simulink model "auto_pilot_udp"  (R2022b)
settings: Solver=FixedStepAuto  StartTime=0.0  StopTime=Inf  FixedStep=0.001  RelTol=1e-3  EnableMultiTasking=on
InitFcn:
  | clear mex
model workspace (MAT data in the model file):
  worldsim_instance : object (value not decoded)
values from neighbouring files (symbols this model uses):
  ACC_Adaptive_D = 0    [AutoPilot_parameters.m]    (also in ap_ini_param.mat; ap_initialModel.sldd = 0.0)
  ACC_Adaptive_I = 0    [AutoPilot_parameters.m]    (also in ap_ini_param.mat; ap_initialModel.sldd = 0.0)
  ACC_Adaptive_P = [5 7.5]    [AutoPilot_parameters.m]    (also in ap_ini_param.mat; ap_initialModel.sldd = 5.0 7.5)
  ACC_Classic_I = 5    [AutoPilot_parameters.m]    (also in ap_ini_param.mat; ap_initialModel.sldd = 5.0)
  ACC_Classic_P = 15    [AutoPilot_parameters.m]    (also in ap_ini_param.mat; ap_initialModel.sldd = 15.0)
  ACC_MaxBrake = 50    [AutoPilot_parameters.m]    (also in ap_ini_param.mat; ap_initialModel.sldd = 50.0)
  ACC_MaxThrottle = 130    [AutoPilot_parameters.m]    (also in ap_ini_param.mat = 80; ap_initialModel.sldd = 130.0)
  ACC_Module_Activity_Flag = 1    [AutoPilot_parameters.m]    (also in ap_ini_param.mat; ap_initialModel.sldd = 1.0)
  ACC_Ready_Speed = 30    [AutoPilot_parameters.m]    (also in ap_ini_param.mat; ap_initialModel.sldd = 30.0)
  ACC_SensorMaxDistance = 250    [AutoPilot_parameters.m]    (also in ap_ini_param.mat = 120; ap_initialModel.sldd = 250.0)
  ACC_Speed_Distance_control = 3    [AutoPilot_parameters.m]    (also in ap_ini_param.mat; ap_initialModel.sldd = 3.0)
  ACC_Speed_Distance_Gain = [0.1 0.15 0.2 0.25]    [AutoPilot_parameters.m]    (also in ap_ini_param.mat; ap_initialModel.sldd = 0.1 0.15 0.2 0.25)
  ADAS_Control_Mode = 1    [AutoPilot_parameters.m]    (also in ap_ini_param.mat; ap_initialModel.sldd = 1.0)
  AEB_Alarm_Freq = 5    [AutoPilot_parameters.m]    (also in ap_ini_param.mat; ap_initialModel.sldd = 5.0)
  AEB_Distance_To_Collision_Brake = 5    [AutoPilot_parameters.m]    (also in ap_ini_param.mat; ap_initialModel.sldd = 5.0)
  AEB_Freq_Hz = Sensor_Freq_worldsim/2    (= 25)    [AutoPilot_parameters.m]    (also in ap_ini_param.mat; ap_initialModel.sldd = 25.0)
  AEB_Gain = [1 1]    [AutoPilot_parameters.m]    (also in ap_ini_param.mat; ap_initialModel.sldd = 1.0 1.0)
  AEB_Gain_set = 60    [AutoPilot_parameters.m]    (also in ap_ini_param.mat; ap_initialModel.sldd = 60.0)
  AEB_Gain_set_mult = 0.03    [AutoPilot_parameters.m]    (also in ap_ini_param.mat; ap_initialModel.sldd)
  AEB_Max_Decel = [8 15]    [AutoPilot_parameters.m]    (also in ap_ini_param.mat; ap_initialModel.sldd = 8.0 15.0)
  AEB_Max_Speed = 150    [AutoPilot_parameters.m]    (also in ap_ini_param.mat = 100; ap_initialModel.sldd = 150.0)
  AEB_Min_Distance_at_Stop = 1    [AutoPilot_parameters.m]    (also in ap_ini_param.mat; ap_initialModel.sldd = 1.0)
  AEB_Module_Activity_Flag = 1    [AutoPilot_parameters.m]    (also in ap_ini_param.mat; ap_initialModel.sldd = 1.0)
  AEB_Pedestrian_type = 68    [AutoPilot_parameters.m]    (also in ap_ini_param.mat; ap_initialModel.sldd = 68.0)
  AEB_Steer_Max = 180    [AutoPilot_parameters.m]    (also in ap_ini_param.mat; ap_initialModel.sldd = 180.0)
  AP_Activity_Flag = 1    [AutoPilot_parameters.m]    (also in ap_ini_param.mat; ap_initialModel.sldd = 1.0)
  AP_D = [0.3 0.3]    [AutoPilot_parameters.m]    (also in ap_ini_param.mat; ap_initialModel.sldd = 0.3 0.3)
  AP_Dyn_Rate_Limiter_Gain = 0.1    [AutoPilot_parameters.m]    (also in ap_ini_param.mat; ap_initialModel.sldd)
  AP_Dyn_Rate_Limiter_Power = 10    [AutoPilot_parameters.m]    (also in ap_ini_param.mat; ap_initialModel.sldd = 10.0)
  AP_Error_Max = 3    [AutoPilot_parameters.m]    (also in ap_ini_param.mat; ap_initialModel.sldd = 3.0)
  AP_Freq_Hz = Sensor_Freq_worldsim    (= 50)    [AutoPilot_parameters.m]    (also in ap_ini_param.mat; ap_initialModel.sldd = 50.0)
  AP_I = [0.05 0.05]    [AutoPilot_parameters.m]    (also in ap_ini_param.mat; ap_initialModel.sldd = 0.05 0.05)
  AP_Max_Error_dydt_Disable = 0.5    [AutoPilot_parameters.m]    (also in ap_ini_param.mat; ap_initialModel.sldd)
  AP_On_Request_Time = 0.01    [AutoPilot_parameters.m]    (also in ap_ini_param.mat; ap_initialModel.sldd)
  AP_P = [0.2 0.2]    [AutoPilot_parameters.m]    (also in ap_ini_param.mat; ap_initialModel.sldd = 0.2 0.2)
  AP_Steer_Error_Max = 0.7    [AutoPilot_parameters.m]    (also in ap_ini_param.mat; ap_initialModel.sldd)
  AP_Steer_Rate_Max_radps = 1    [AutoPilot_parameters.m]    (also in ap_ini_param.mat; ap_initialModel.sldd = 1.0)
  AP_Transition_Rate = 0.5    [AutoPilot_parameters.m]    (also in ap_ini_param.mat; ap_initialModel.sldd)
  butter_a = [1 -1.9911142922 0.991153595869]    [ap_ini_param.mat]    (also in ap_initialModel.sldd = 1.0 -1.9911142922016536 0.99115359586893548)
  butter_a_lka_out = 1.0 -1.5610180758007179 0.641351538057563    [ap_initialModel.sldd]
  butter_b = [9.82591682048e-06 1.9651833641e-05 9.82591682048e-06]    [ap_ini_param.mat]    (also in ap_initialModel.sldd = 9.825916820482009E-6 1.9651833640964018E-5 9.825916820482009)
  butter_b_lka_out = 0.020083365564211246 0.040166731128422492 0.020083365564211246    [ap_initialModel.sldd]
  Lane_Width = 3.7    [AutoPilot_parameters.m]    (also in ap_ini_param.mat; ap_initialModel.sldd)
  LDW_Activity_Flag = 1    [ap_ini_param.mat]    (also in ap_initialModel.sldd = 1.0)
  LDW_Freq_Hz = 50    [ap_ini_param.mat]    (also in ap_initialModel.sldd = 50.0)
  LDW_LaneGap_dydt_Warning = 50    [ap_ini_param.mat]    (also in ap_initialModel.sldd = 50.0)
  LDW_LaneGap_Warning = [0.5 0.25]    [ap_ini_param.mat]    (also in ap_initialModel.sldd = 0.5 0.25)
  LDW_Min_Speed = 60    [ap_ini_param.mat]    (also in ap_initialModel.sldd = 60.0)
  LDW_Steer_Vibration_Amplitude = 5    [ap_ini_param.mat]    (also in ap_initialModel.sldd = 5.0)
  LDW_Steer_Vibration_Freq = 25    [ap_ini_param.mat]    (also in ap_initialModel.sldd = 25.0)
  LKA_Activity_Flag = 1    [ap_ini_param.mat]    (also in ap_initialModel.sldd = 1.0)
  LKA_D = [0.2 0.3]    [ap_ini_param.mat]    (also in ap_initialModel.sldd = 0.2 0.3)
  LKA_Dyn_Rate_Limiter_Gain = 0.1    [ap_ini_param.mat]    (also in ap_initialModel.sldd)
  LKA_Dyn_Rate_Limiter_Power = 10    [ap_ini_param.mat]    (also in ap_initialModel.sldd = 10.0)
  LKA_Error_dydt_Off = 1    [ap_ini_param.mat]    (also in ap_initialModel.sldd = 1.0)
  LKA_Error_Max = 3    [ap_ini_param.mat]    (also in ap_initialModel.sldd = 3.0)
  LKA_Error_Off = 0.5    [ap_ini_param.mat]    (also in ap_initialModel.sldd)
  LKA_Freq_Hz = 50    [ap_ini_param.mat]    (also in ap_initialModel.sldd = 50.0)
  LKA_I = [0.025 0.05]    [ap_ini_param.mat]    (also in ap_initialModel.sldd = 0.025 0.05)
  LKA_Lane_Gap_Activate = [0.25 0.125]    [ap_ini_param.mat]    (also in ap_initialModel.sldd = 0.25 0.125)
  LKA_Lane_Gap_dydt_Activate = 50    [ap_ini_param.mat]    (also in ap_initialModel.sldd = 50.0)
  LKA_Min_Speed = 60    [ap_ini_param.mat]    (also in ap_initialModel.sldd = 60.0)
  LKA_On_Display_Freq = 5    [ap_ini_param.mat]    (also in ap_initialModel.sldd = 5.0)
  LKA_P = [0.1 0.2]    [ap_ini_param.mat]    (also in ap_initialModel.sldd = 0.1 0.2)
  LKA_Steer_Rate_Max_radps = 1    [ap_ini_param.mat]    (also in ap_initialModel.sldd = 1.0)
  No_Target_Display_Value = 0    [AutoPilot_parameters.m]    (also in ap_ini_param.mat; ap_initialModel.sldd = 0.0)
  radar_source = 2    [AutoPilot_parameters.m]    (also in ap_ini_param.mat; ap_initialModel.sldd = 2.0)
  Sensor_Freq_worldsim = 50    [AutoPilot_parameters.m]    (also in ap_ini_param.mat; ap_initialModel.sldd = 50.0; launcher.m)
  stop_number_collisions = 10.0    [ap_initialModel.sldd]    (also in launcher.m = 10)
  stop_speed = 0.001    [ap_initialModel.sldd]    (also in launcher.m)
  stop_time = 12.0    [ap_initialModel.sldd]    (also in launcher.m = 12)
  vehicle_width = 2.2    [AutoPilot_parameters.m]    (also in ap_ini_param.mat = 1.86; ap_initialModel.sldd)
undefined symbols (not defined in the file or in its folder): blockPlatform, HOST, light_brake_center, light_brake_left, light_brake_right
libraries: simulink x103, simwbSfunlib x35, slpidlib x5, viworldsim_lib x5
(part 3 of 5)

== system auto_pilot_udp/OUTPUT/VI-CarRealTime_Outputs2 ==
  Constant : Constant  Value=0
  Gain : Gain  Gain=1/2
  Log_Bus_Creator : BusCreator  Inputs=9
  Log_bus : BusSelector  OutputSignals=VI_CarRealTime:Outputs:chassis_velocities:longitudinal,VI_CarRealTime:Outputs:driver_demands:steering,VI_CarRealTime:Outputs:Wheel:Spindle_Steer:L1,VI_CarRealTime:Outputs:Wheel:Spindle_Steer:R1,VI_CarRealTime:Outputs:driver_demands:throttle,VI_CarRealTime:Outputs:driver_demands:brake,VI_CarRealTime:Outputs:chassis_accelerations:longitudinal,VI_CarRealTime:Outputs:chassis_accelerations:lateral,VI_CarRealTime:Outputs:Steering_System:DriveSim_Steering_Feedback_Torque  OutputAsBus=on
  Scope : Scope  NumInputPorts=2
  Sum : Sum
  Terminator : Terminator
  Terminator1 : Terminator
  VI_CarRealTime.Outputs.Steering_System.DriveSim_Steering_Feedback_Torque : simwbSfunlib/fromRTDBm  varName=VI_CarRealTime.Outputs.Steering_System.DriveSim_Steering_Feedback_Torque  sigDim=[1 1]  sigType=double  sampleTime=[-1 0]  defaultValue=0  hasMapping=0  ptrName=VI_CarRealTime_Outputs_chassis_accelerations_lateral  enumOrAlias=nothing
      settings: SourceProductName=SimWB MLToolkit
  VI_CarRealTime.Outputs.Wheel.Spindle_Steer.L1 : simwbSfunlib/fromRTDBm  varName=VI_CarRealTime.Outputs.Wheel.Spindle_Steer.L1  sigDim=[1 1]  sigType=double  sampleTime=[-1 0]  defaultValue=0  hasMapping=0  ptrName=VI_CarRealTime_Outputs_Wheel_Spindle_Steer_L1  enumOrAlias=nothing
      settings: SourceProductName=SimWB MLToolkit
  VI_CarRealTime.Outputs.Wheel.Spindle_Steer.R1 : simwbSfunlib/fromRTDBm  varName=VI_CarRealTime.Outputs.Wheel.Spindle_Steer.R1  sigDim=[1 1]  sigType=double  sampleTime=[-1 0]  defaultValue=0  hasMapping=0  ptrName=VI_CarRealTime_Outputs_Wheel_Spindle_Steer_R1  enumOrAlias=nothing
      settings: SourceProductName=SimWB MLToolkit
  VI_CarRealTime.Outputs.chassis_accelerations.lateral : simwbSfunlib/fromRTDBm  varName=VI_CarRealTime.Outputs.chassis_accelerations.lateral  sigDim=[1 1]  sigType=double  sampleTime=[-1 0]  defaultValue=0  hasMapping=0  ptrName=VI_CarRealTime_Outputs_chassis_accelerations_longitudinal  enumOrAlias=nothing
      settings: SourceProductName=SimWB MLToolkit
  VI_CarRealTime.Outputs.chassis_accelerations.longitudinal : simwbSfunlib/fromRTDBm  varName=VI_CarRealTime.Outputs.chassis_accelerations.longitudinal  sigDim=[1 1]  sigType=double  sampleTime=[-1 0]  defaultValue=0  hasMapping=0  ptrName=VI_CarRealTime_Outputs_chassis_velocities_longitudinal  enumOrAlias=nothing
      settings: SourceProductName=SimWB MLToolkit
  VI_CarRealTime.Outputs.chassis_velocities.longitudinal : simwbSfunlib/fromRTDBm  varName=VI_CarRealTime.Outputs.chassis_velocities.longitudinal  sigDim=[1 1]  sigType=double  sampleTime=[-1 0]  defaultValue=0  hasMapping=0  ptrName=VI_CarRealTime_Outputs_chassis_velocities_longitudinal  enumOrAlias=nothing
      settings: SourceProductName=SimWB MLToolkit
  VI_CarRealTime.Outputs.driver_demands.brake : simwbSfunlib/fromRTDBm  varName=VI_CarRealTime.Outputs.driver_demands.brake  sigDim=[1 1]  sigType=double  sampleTime=[-1 0]  defaultValue=0  hasMapping=0  ptrName=VI_CarRealTime_Outputs_driver_demands_throttle  enumOrAlias=nothing
      settings: SourceProductName=SimWB MLToolkit
  VI_CarRealTime.Outputs.driver_demands.steering : simwbSfunlib/fromRTDBm  varName=VI_CarRealTime.Outputs.driver_demands.steering  sigDim=[1 1]  sigType=double  sampleTime=[-1 0]  defaultValue=0  hasMapping=0  ptrName=VI_CarRealTime_Outputs_chassis_velocities_longitudinal  enumOrAlias=nothing
      settings: SourceProductName=SimWB MLToolkit
  VI_CarRealTime.Outputs.driver_demands.throttle : simwbSfunlib/fromRTDBm  varName=VI_CarRealTime.Outputs.driver_demands.throttle  sigDim=[1 1]  sigType=double  sampleTime=[-1 0]  defaultValue=0  hasMapping=0  ptrName=VI_CarRealTime_Outputs_driver_demands_steering  enumOrAlias=nothing
      settings: SourceProductName=SimWB MLToolkit
  tag scope: Driver_Brake=global, Driver_Steering=global, Driver_Throttle=global, Front_Axle_Steer=global, Lateral_Accelerations=global, Longitudinal_Accelerations=global, Steering_feedback_torque=global, Vehicle_Speed=global
  wires:
  ? -> Scope/1, [Vehicle_Speed]
  Log_bus/1 -> Terminator/1  "VI_CarRealTime_selection"
  ? -> Scope/2, [Driver_Steering]
  ? -> Sum/1
  ? -> Sum/2
  Sum/1 -> Gain/1
  Gain/1 -> [Front_Axle_Steer]
  ? -> [Driver_Throttle]
  Constant/1 -> [Driver_Brake]
  ? -> Terminator1/1
  ? -> [Longitudinal_Accelerations]
  ? -> [Lateral_Accelerations]
  ? -> [Steering_feedback_torque]
  VI_CarRealTime.Outputs.driver_demands.brake/1 -> Log_Bus_Creator/6  "VI_CarRealTime.Outputs.driver_demands.brake"
  VI_CarRealTime.Outputs.Wheel.Spindle_Steer.L1/1 -> Log_Bus_Creator/3  "VI_CarRealTime.Outputs.Wheel.Spindle_Steer.L1"
  VI_CarRealTime.Outputs.chassis_accelerations.lateral/1 -> Log_Bus_Creator/8  "VI_CarRealTime.Outputs.chassis_accelerations.lateral"
  VI_CarRealTime.Outputs.Steering_System.DriveSim_Steering_Feedback_Torque/1 -> Log_Bus_Creator/9  "VI_CarRealTime.Outputs.Steering_System.DriveSim_Steering_Feedback_Torque"
  VI_CarRealTime.Outputs.chassis_accelerations.longitudinal/1 -> Log_Bus_Creator/7  "VI_CarRealTime.Outputs.chassis_accelerations.longitudinal"
  VI_CarRealTime.Outputs.driver_demands.steering/1 -> Log_Bus_Creator/2  "VI_CarRealTime.Outputs.driver_demands.steering"
  VI_CarRealTime.Outputs.Wheel.Spindle_Steer.R1/1 -> Log_Bus_Creator/4  "VI_CarRealTime.Outputs.Wheel.Spindle_Steer.R1"
  VI_CarRealTime.Outputs.driver_demands.throttle/1 -> Log_Bus_Creator/5  "VI_CarRealTime.Outputs.driver_demands.throttle"
  VI_CarRealTime.Outputs.chassis_velocities.longitudinal/1 -> Log_Bus_Creator/1  "VI_CarRealTime.Outputs.chassis_velocities.longitudinal"
  Log_Bus_Creator/1 -> Log_bus/1

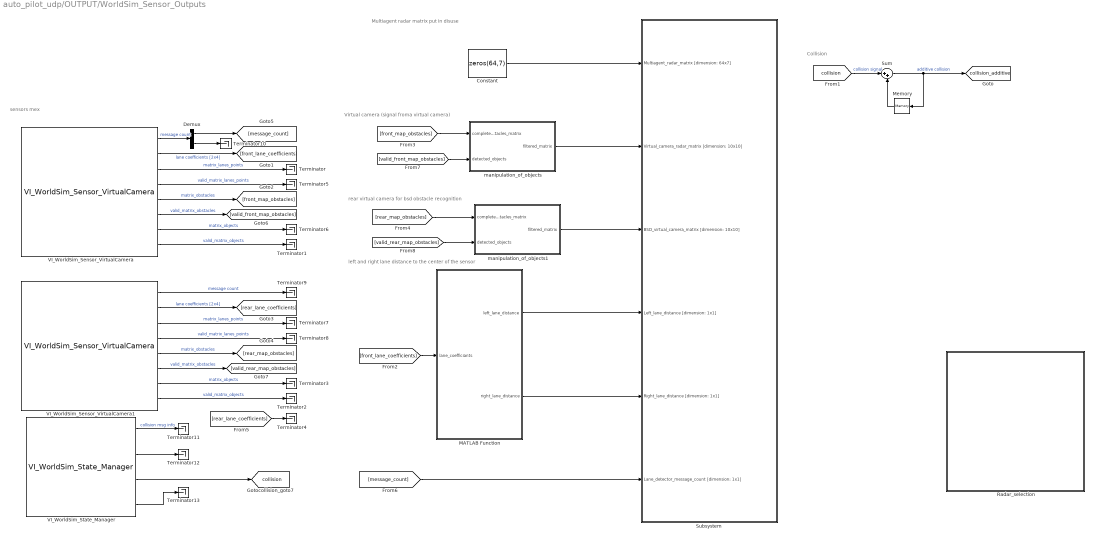
== system auto_pilot_udp/OUTPUT/WorldSim_Sensor_Outputs ==
  note: Collision
  note: left and right lane distance to the center of the sensor
  note: Virtual camera (signal froma virtual camera)
  note: Multiagent radar matrix
      | put in disuse
  note: rear virtual camera for bsd obstacle recognition
  note: sensors mex
  Constant : Constant  Value=zeros(64,7)
  Demux : Demux  Outputs=2
  MATLAB Function : MATLAB Function  TreatAsAtomicUnit=on
  Memory : Memory  InheritSampleTime=on
  Radar_selection : Subsystem
  Subsystem : Subsystem
  Sum : Sum  Inputs=|++
  Terminator{,1..13} (14 alike) : Terminator
  VI_WorldSim_Sensor_VirtualCamera : viworldsim_lib/VI-WorldSim Sensors/VI_WorldSim_Sensor_VirtualCamera  worldsim_endpoint_ip=worldsim_instance.endpoint_ip  worldsim_endpoint_port=worldsim_instance.endpoint_port  worldsim_car_name='ego'  worldsim_sensor_name='Front_VirtualCam'  max_lanes=10  max_obstacles=10  worldsim_verbose=off
  VI_WorldSim_Sensor_VirtualCamera1 : viworldsim_lib/VI-WorldSim Sensors/VI_WorldSim_Sensor_VirtualCamera  worldsim_endpoint_ip=worldsim_instance.endpoint_ip  worldsim_endpoint_port=worldsim_instance.endpoint_port  worldsim_car_name='ego'  worldsim_sensor_name='Rear_VirtualCam'  max_lanes=10  max_obstacles=10  worldsim_verbose=off
  VI_WorldSim_State_Manager : viworldsim_lib/VI-WorldSim Sensors/VI_WorldSim_State_Manager  worldsim_endpoint_ip=worldsim_instance.endpoint_ip  worldsim_endpoint_port=worldsim_instance.endpoint_port  worldsim_car_name='ego'  worldsim_verbose=off
  manipulation_of_objects : MATLAB Function  TreatAsAtomicUnit=on
  manipulation_of_objects1 : MATLAB Function  TreatAsAtomicUnit=on
  tag scope: collision=global, collision_additive=global
  wires:
  Sum/1 -> Memory/1, [collision_additive]  "additive collision"
  [collision] -> Sum/1  "collision signal"
  Memory/1 -> Sum/2
  MATLAB Function/1(left_lane_distance) -> Subsystem/4(Left_lane_distance [dimension: 1x1])
  [message_count] -> Subsystem/6(Lane_detector_message_count [dimension: 1x1])
  manipulation_of_objects1/1(filtered_matrix) -> Subsystem/3(BSD_virtual_camera_matrix [dimension: 10x10])
  manipulation_of_objects/1(filtered_matrix) -> Subsystem/2(Virtual_camera_radar_matrix [dimension: 10x10])
  Constant/1 -> Subsystem/1(Multiagent_radar_matrix [dimension: 64x7])
  [valid_rear_map_obstacles] -> manipulation_of_objects1/2(detected_objects)
  MATLAB Function/2(right_lane_distance) -> Subsystem/5(Right_lane_distance [dimension: 1x1])
  [front_lane_coefficients] -> MATLAB Function/1(lane_coefficiants)
  [rear_map_obstacles] -> manipulation_of_objects1/1(complete_obstacles_matrix)
  [valid_front_map_obstacles] -> manipulation_of_objects/2(detected_objects)
  [front_map_obstacles] -> manipulation_of_objects/1(complete_obstacles_matrix)
  VI_WorldSim_Sensor_VirtualCamera/1 -> Demux/1  "message count"
  VI_WorldSim_State_Manager/1 -> Terminator11/1  "collision msg info"
  VI_WorldSim_Sensor_VirtualCamera/8 -> Terminator1/1  "valid_matrix_objects"
  VI_WorldSim_Sensor_VirtualCamera/5 -> [front_map_obstacles]  "matrix_obstacles"
  VI_WorldSim_Sensor_VirtualCamera/4 -> Terminator5/1  "valid_matrix_lanes_points"
  VI_WorldSim_Sensor_VirtualCamera/6 -> [valid_front_map_obstacles]  "valid_matrix_obstacles"
  VI_WorldSim_Sensor_VirtualCamera1/2 -> [rear_lane_coefficients]  "lane coefficients [2x4]"
  VI_WorldSim_Sensor_VirtualCamera/3 -> Terminator/1  "matrix_lanes_points"
  VI_WorldSim_Sensor_VirtualCamera1/1 -> Terminator9/1  "message count"
  VI_WorldSim_Sensor_VirtualCamera1/7 -> Terminator3/1  "matrix_objects"
  VI_WorldSim_Sensor_VirtualCamera1/8 -> Terminator2/1  "valid_matrix_objects"
  VI_WorldSim_Sensor_VirtualCamera/7 -> Terminator6/1  "matrix_objects"
  VI_WorldSim_Sensor_VirtualCamera/2 -> [front_lane_coefficients]  "lane coefficients [2x4]"
  VI_WorldSim_Sensor_VirtualCamera1/4 -> Terminator8/1  "valid_matrix_lanes_points"
  VI_WorldSim_State_Manager/3 -> [collision]
  VI_WorldSim_Sensor_VirtualCamera1/3 -> Terminator7/1  "matrix_lanes_points"
  [rear_lane_coefficients] -> Terminator4/1
  Demux/2 -> Terminator10/1
  VI_WorldSim_Sensor_VirtualCamera1/5 -> [rear_map_obstacles]  "matrix_obstacles"
  VI_WorldSim_Sensor_VirtualCamera1/6 -> [valid_rear_map_obstacles]  "valid_matrix_obstacles"
  Demux/1 -> [message_count]
  VI_WorldSim_State_Manager/2 -> Terminator12/1
  VI_WorldSim_State_Manager/4 -> Terminator13/1

== system auto_pilot_udp/OUTPUT/rough data reporting ==
  Cast To Double : DataTypeConversion  OutDataTypeStr=double  SaturateOnIntegerOverflow=off  RndMeth=Floor
  Cast To Double1 : DataTypeConversion  OutDataTypeStr=double  SaturateOnIntegerOverflow=off  RndMeth=Floor
  Clock : Clock
  Compare To Constant : simulink/Logic and Bit Operations/Compare To Constant  relop=<=  const=0.0  OutDataTypeStr=boolean
  Compare To Constant1 : simulink/Logic and Bit Operations/Compare To Constant  relop=<=  const=0.0  OutDataTypeStr=boolean
  Compare To Constant2 : simulink/Logic and Bit Operations/Compare To Constant  relop=>  const=0.1  OutDataTypeStr=boolean
  Constant : Constant  Value=0
  Mux : Mux  Inputs=2
  Product : Product
  Scope LDW_Steering_Torque_in_out : Scope
  Sum1 : Sum
  To Workspace : ToWorkspace  VariableName=number_collision  SampleTime=-1
      settings: Save2DSignal=2-D array (concatenate along first dimension)
  To Workspace1 : ToWorkspace  VariableName=longitudinal_accelerations  SampleTime=-1
      settings: Save2DSignal=2-D array (concatenate along first dimension)
  To Workspace2 : ToWorkspace  VariableName=lateral_accelerations  SampleTime=-1
      settings: Save2DSignal=2-D array (concatenate along first dimension)
  To Workspace3 : ToWorkspace  VariableName=crossed_lanes  SampleTime=-1
      settings: Save2DSignal=2-D array (concatenate along first dimension)
  wires:
  Clock/1 -> Compare To Constant2/1
  Compare To Constant1/1 -> Cast To Double1/1
  [Lateral_Accelerations] -> To Workspace2/1
  [LaneGap_right_ws] -> Compare To Constant1/1
  Cast To Double/1 -> Sum1/1
  Compare To Constant2/1 -> Product/2
  [collision_additive] -> To Workspace/1
  Compare To Constant/1 -> Cast To Double/1
  [Longitudinal_Accelerations] -> To Workspace1/1
  [LaneGap_left_ws] -> Compare To Constant/1
  Product/1 -> To Workspace3/1
  Cast To Double1/1 -> Sum1/2
  Sum1/1 -> Product/1
  [Steering_feedback_torque] -> Mux/2
  [LDW_Steering_Torque] -> Mux/1
  Mux/1 -> Scope LDW_Steering_Torque_in_out/1  "LDW_Steering_Torque_in_out"
  Constant/1 -> [LDW_Steering_Torque]

== system auto_pilot_udp/VI-WorldSim Lights Manager/Lights ==
  light_brake_left : Inport
  light_brake_right : Inport  Port=2
  light_brake_center : Inport  Port=3
  Bus Selector : BusSelector  OutputSignals=light_low_beam_left,light_low_beam_right,light_high_beam_left,light_high_beam_right,light_indicator_left,light_indicator_right,light_fog_left,light_fog_right,light_tail_left,light_tail_right,light_brake_left,light_brake_right,light_brake_center,light_reverse,light_daytime
  Default Lights Bus : Subsystem
  LightsBusAssignment : BusAssignment  AssignedSignals=light_brake_left,light_brake_right,light_brake_center
  Mux : Mux  Inputs=15
  Out1 : Outport  VectorParamsAs1DForOutWhenUnconnected=off
  wires:
  LightsBusAssignment/1 -> Bus Selector/1
  Bus Selector/5 -> Mux/5  "<light_indicator_left>"
  Default Lights Bus/1(Out1) -> LightsBusAssignment/1
  Bus Selector/11 -> Mux/11  "<light_brake_left>"
  Bus Selector/10 -> Mux/10  "<light_tail_right>"
  Bus Selector/2 -> Mux/2  "<light_low_beam_right>"
  Bus Selector/9 -> Mux/9  "<light_tail_left>"
  Bus Selector/12 -> Mux/12  "<light_brake_right>"
  Mux/1 -> Out1/1
  Bus Selector/8 -> Mux/8  "<light_fog_right>"
  Bus Selector/14 -> Mux/14  "<light_reverse>"
  Bus Selector/4 -> Mux/4  "<light_high_beam_right>"
  Bus Selector/3 -> Mux/3  "<light_high_beam_left>"
  Bus Selector/15 -> Mux/15  "<light_daytime>"
  Bus Selector/13 -> Mux/13  "<light_brake_center>"
  Bus Selector/6 -> Mux/6  "<light_indicator_right>"
  Bus Selector/1 -> Mux/1  "<light_low_beam_left>"
  Bus Selector/7 -> Mux/7  "<light_fog_left>"
  light_brake_left/1 -> LightsBusAssignment/2
  light_brake_right/1 -> LightsBusAssignment/3
  light_brake_center/1 -> LightsBusAssignment/4

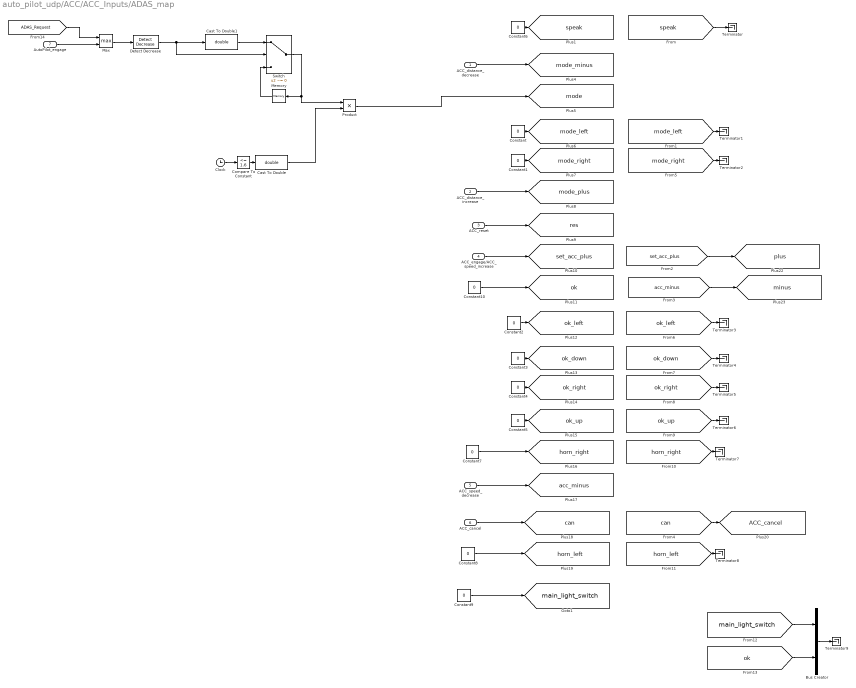
== system auto_pilot_udp/ACC/ACC_Inputs/ADAS_map ==
  ACC_distance_decrease : Inport
  ACC_distance_increase : Inport  Port=2
  ACC_reset : Inport  Port=3
  ACC_engage/ACC_speed_increase : Inport  Port=4
  ACC_speed_decrease : Inport  Port=5
  ACC_cancel : Inport  Port=6
  AutoPilot_engage : Inport  Port=7
  Bus Creator : BusCreator  Inputs=2
  Cast To Double : DataTypeConversion  OutDataTypeStr=double  SaturateOnIntegerOverflow=off  RndMeth=Floor
  Cast To Double1 : DataTypeConversion  OutDataTypeStr=double  SaturateOnIntegerOverflow=off  RndMeth=Floor
  Clock : Clock
  Compare To Constant : simulink/Logic and Bit Operations/Compare To Constant  relop=<=  const=1.6  OutDataTypeStr=boolean
  Constant{,1..10} (11 alike) : Constant  Value=0
  Detect Decrease : simulink/Logic and Bit Operations/Detect Decrease  vinit=0.0  OutDataTypeStr=boolean
  Max : MinMax  Function=max  Inputs=2
  Memory : Memory  InheritSampleTime=on
  Product : Product
  Switch : Switch  Criteria=u2 ~= 0  SaturateOnIntegerOverflow=off  InputSameDT=off
  Terminator{,1..9} (10 alike) : Terminator
  tag scope: ACC_cancel=global, acc_minus=global, can=global, horn_left=global, horn_right=global, main_light_switch=global, minus=global, mode=global, mode_left=global, mode_minus=global, mode_plus=global, mode_right=global, ok=global, ok_down=global, ok_left=global, ok_right=global, ok_up=global, plus=global, res=global, set_acc_plus=global, speak=global
  wires:
  [set_acc_plus] -> [plus]
  ACC_speed_decrease/1 -> [acc_minus]
  Constant10/1 -> [ok]
  Constant8/1 -> [horn_left]
  [acc_minus] -> [minus]
  ACC_engage/ACC_speed_increase/1 -> [set_acc_plus]
  ACC_reset/1 -> [res]
  ACC_cancel/1 -> [can]
  ACC_distance_increase/1 -> [mode_plus]
  ACC_distance_decrease/1 -> [mode_minus]
  Constant7/1 -> [horn_right]
  Constant6/1 -> [speak]
  [can] -> [ACC_cancel]
  Constant9/1 -> [main_light_switch]
  Constant/1 -> [mode_left]
  Constant1/1 -> [mode_right]
  Constant2/1 -> [ok_left]
  Constant3/1 -> [ok_down]
  Constant4/1 -> [ok_right]
  Constant5/1 -> [ok_up]
  [speak] -> Terminator/1
  [mode_left] -> Terminator1/1
  [mode_right] -> Terminator2/1
  [ok_left] -> Terminator3/1
  [ok_down] -> Terminator4/1
  [ok_right] -> Terminator5/1
  [ok_up] -> Terminator6/1
  [horn_right] -> Terminator7/1
  [horn_left] -> Terminator8/1
  Switch/1 -> Product/1, Memory/1
  Memory/1 -> Switch/3
  Clock/1 -> Compare To Constant/1
  Compare To Constant/1 -> Cast To Double/1
  Cast To Double/1 -> Product/2
  Product/1 -> [mode]
  [main_light_switch] -> Bus Creator/1
  [ok] -> Bus Creator/2
  Bus Creator/1 -> Terminator9/1
  Detect Decrease/1 -> Switch/2, Cast To Double1/1
  Cast To Double1/1 -> Switch/1
  Max/1 -> Detect Decrease/1
  [ADAS_Request] -> Max/1
  AutoPilot_engage/1 -> Max/2

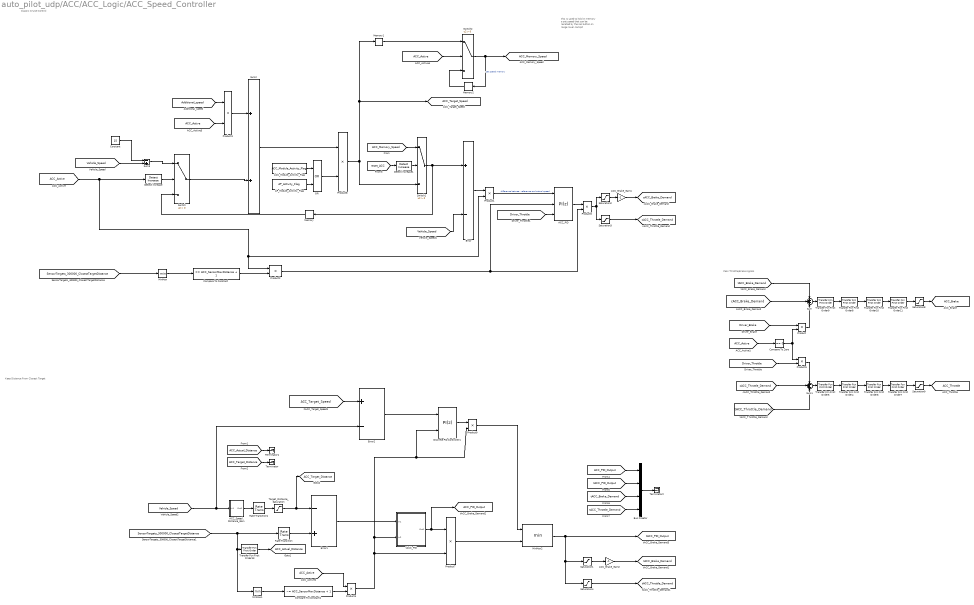
== system auto_pilot_udp/ACC/ACC_Logic/ACC_Speed_Controller ==
  note: this is used to hold in memory a set speed that can be recalled by the res button on range rover cockpit
  note: Pass Throttle/Brake signals
  note: Keep Distance From Closest Target
  note: Classic Cruise Control
  ACC_Brake_Gain1 : Gain  Gain=-1
  ACC_Brake_Gain2 : Gain  Gain=-1
  ACC_Module_Activity_Flag : Constant  Value=ACC_Module_Activity_Flag
  ACC_PID : slpidlib/PID Controller  Controller=PI  Form=Parallel  TimeDomain=Discrete-time  UseExternalTs=off  SampleTime=-1  IntegratorMethod=Forward Euler  FilterMethod=Forward Euler  ControllerParametersSource=internal  P=ACC_Classic_P  I=ACC_Classic_I  UseKiTs=off  D=0  N=100  UseFilter=on  TunerSelectOption=Transfer Function Based (PID Tuner App)  InitialConditionSource=external  InitialConditionForIntegrator=0  InitialConditionForFilter=0  DifferentiatorICPrevScaledInput=0  ExternalReset=either  TrackingMode=off  Kt=1  LimitOutput=on  SatLimitsSource=internal  UpperSaturationLimit=ACC_MaxThrottle  LowerSaturationLimit=-ACC_MaxBrake  LinearizeAsGain=off  AntiWindupMode=back-calculation  Kb=1  LimitIntegrator=off  UpperIntegratorSaturationLimit=inf  LowerIntegratorSaturationLimit=-inf  POutMin=[]  POutMax=[]  IOutMin=[]  IOutMax=[]  DOutMin=[]  DOutMax=[]  NOutMin=[]  NOutMax=[]  SumOutMin=[]  SumOutMax=[]  SaturationOutMin=[]  SaturationOutMax=[]  PParamMin=[]  PParamMax=[]  IParamMin=[]  IParamMax=[]  DParamMin=[]  DParamMax=[]  NParamMin=[]  NParamMax=[]  KbParamMin=[]  KbParamMax=[]  KtParamMin=[]  KtParamMax=[]  KbOutMin=[]  KbOutMax=[]  KtOutMin=[]  KtOutMax=[]  IntegratorOutMin=[]  IntegratorOutMax=[]  FilterOutMin=[]  FilterOutMax=[]  SumI1OutMin=[]  SumI1OutMax=[]  SumI2OutMin=[]  SumI2OutMax=[]  SumI3OutMin=[]  SumI3OutMax=[]  SumI4OutMin=[]  SumI4OutMax=[]  SumDOutMin=[]  SumDOutMax=[]  DifferentiatorOutMin=[]  DifferentiatorOutMax=[]  FilterDiffOutCoefMin=[]  FilterDiffOutCoefMax=[]  ReciprocalOutMin=[]  ReciprocalOutMax=[]  SumDenOutMin=[]  SumDenOutMax=[]  SumNumOutMin=[]  SumNumOutMax=[]  DivideOutMin=[]  DivideOutMax=[]  UdiffTsProdOutMin=[]  UdiffTsProdOutMax=[]  NTsProdOutMin=[]  NTsProdOutMax=[]  UintegralTsProdOutMin=[]  UintegralTsProdOutMax=[]  UngainTsProdOutMin=[]  UngainTsProdOutMax=[]  ClampingZeroOutDataTypeStr=Inherit: Inherit via back propagation  ClampingZeroOutMin=[]  ClampingZeroOutMax=[]  FilterDenConstantOutDataTypeStr=Inherit: Inherit via back propagation  FilterDenConstantOutMin=[]  FilterDenConstantOutMax=[]  PCopyOutDataTypeStr=Inherit: Inherit via back propagation  PCopyOutMin=[]  PCopyOutMax=[]  NCopyOutDataTypeStr=Inherit: Inherit via back propagation  NCopyOutMin=[]  NCopyOutMax=[]  IntegratorContinuousStateAttributes=''  IntegratorStateMustResolveToSignalObject=off  IntegratorRTWStateStorageClass=Auto  FilterContinuousStateAttributes=''  FilterStateMustResolveToSignalObject=off  FilterRTWStateStorageClass=Auto  ParallelPVariant=InternalParameters  IdealPVariant=Disabled  IVariant=InternalParameters  DVariant=Disabled  IntegratorVariant=Discrete  SatVariant=Enabled  AWVariant=BackCalculation  PCopyVariant=Disabled  TRVariant=Disabled  FdbkBlocksVariant=Forward  IdealPFdbkVariant=Disabled  SatFdbkVariant=Disabled  DerivativeFilterVariant=Disabled  NVariant=Disabled  NCopyVariant=Disabled_SignalSpec  FilterICVariant=Disabled  IntegratorICVariant=ExternalICs  ExternalResetVariant=ExternalReset  TRSumVariant=Passthrough  SumFdbkVariant=Disabled  SumVariant=Sum_PI  TsampFilterVariant=InternalTs  TsampNgainVariant=Passthrough  TsampIntegralVariant=Passthrough  ExternalSaturationOutDataTypeStr=Inherit: Same as second input
  ACC_Speed_Distance_Gain : Subsystem
  AP_Module_Activity_Flag : Constant  Value=AP_Activity_Flag
  Bus Creator : BusCreator  Inputs=4
  Compare To Constant : simulink/Logic and Bit Operations/Compare To Constant  relop===  const=ACC_SensorMaxDistance + 1  OutDataTypeStr=boolean
  Compare To Constant1 : simulink/Logic and Bit Operations/Compare To Constant  relop=~=  const=ACC_SensorMaxDistance + 1  OutDataTypeStr=boolean
  Compare To Zero : simulink/Logic and Bit Operations/Compare To Zero  relop===  OutDataTypeStr=boolean
  Constant : Constant  Value=15
  Detect Increase : simulink/Logic and Bit Operations/Detect Increase  vinit=0.0  OutDataTypeStr=boolean
  Detect Increase1 : simulink/Logic and Bit Operations/Detect Increase  vinit=0.0  OutDataTypeStr=boolean
  Discrete PID Controller1 : slpidlib/PID Controller  Controller=PI  Form=Parallel  TimeDomain=Discrete-time  UseExternalTs=off  SampleTime=-1  IntegratorMethod=Forward Euler  FilterMethod=Forward Euler  ControllerParametersSource=internal  P=ACC_Classic_P  I=ACC_Classic_I  UseKiTs=off  D=0  N=100  UseFilter=on  TunerSelectOption=Transfer Function Based (PID Tuner App)  InitialConditionSource=internal  InitialConditionForIntegrator=0  InitialConditionForFilter=0  DifferentiatorICPrevScaledInput=0  ExternalReset=either  TrackingMode=off  Kt=1  LimitOutput=on  SatLimitsSource=internal  UpperSaturationLimit=ACC_MaxThrottle  LowerSaturationLimit=-ACC_MaxBrake  LinearizeAsGain=off  AntiWindupMode=back-calculation  Kb=1  LimitIntegrator=off  UpperIntegratorSaturationLimit=inf  LowerIntegratorSaturationLimit=-inf  POutMin=[]  POutMax=[]  IOutMin=[]  IOutMax=[]  DOutMin=[]  DOutMax=[]  NOutMin=[]  NOutMax=[]  SumOutMin=[]  SumOutMax=[]  SaturationOutMin=[]  SaturationOutMax=[]  PParamMin=[]  PParamMax=[]  IParamMin=[]  IParamMax=[]  DParamMin=[]  DParamMax=[]  NParamMin=[]  NParamMax=[]  KbParamMin=[]  KbParamMax=[]  KtParamMin=[]  KtParamMax=[]  KbOutMin=[]  KbOutMax=[]  KtOutMin=[]  KtOutMax=[]  IntegratorOutMin=[]  IntegratorOutMax=[]  FilterOutMin=[]  FilterOutMax=[]  SumI1OutMin=[]  SumI1OutMax=[]  SumI2OutMin=[]  SumI2OutMax=[]  SumI3OutMin=[]  SumI3OutMax=[]  SumI4OutMin=[]  SumI4OutMax=[]  SumDOutMin=[]  SumDOutMax=[]  DifferentiatorOutMin=[]  DifferentiatorOutMax=[]  FilterDiffOutCoefMin=[]  FilterDiffOutCoefMax=[]  ReciprocalOutMin=[]  ReciprocalOutMax=[]  SumDenOutMin=[]  SumDenOutMax=[]  SumNumOutMin=[]  SumNumOutMax=[]  DivideOutMin=[]  DivideOutMax=[]  UdiffTsProdOutMin=[]  UdiffTsProdOutMax=[]  NTsProdOutMin=[]  NTsProdOutMax=[]  UintegralTsProdOutMin=[]  UintegralTsProdOutMax=[]  UngainTsProdOutMin=[]  UngainTsProdOutMax=[]  ClampingZeroOutDataTypeStr=Inherit: Inherit via back propagation  ClampingZeroOutMin=[]  ClampingZeroOutMax=[]  FilterDenConstantOutDataTypeStr=Inherit: Inherit via back propagation  FilterDenConstantOutMin=[]  FilterDenConstantOutMax=[]  PCopyOutDataTypeStr=Inherit: Inherit via back propagation  PCopyOutMin=[]  PCopyOutMax=[]  NCopyOutDataTypeStr=Inherit: Inherit via back propagation  NCopyOutMin=[]  NCopyOutMax=[]  IntegratorContinuousStateAttributes=''  IntegratorStateMustResolveToSignalObject=off  IntegratorRTWStateStorageClass=Auto  FilterContinuousStateAttributes=''  FilterStateMustResolveToSignalObject=off  FilterRTWStateStorageClass=Auto  ParallelPVariant=InternalParameters  IdealPVariant=Disabled  IVariant=InternalParameters  DVariant=Disabled  IntegratorVariant=Discrete  SatVariant=Enabled  AWVariant=BackCalculation  PCopyVariant=Disabled  TRVariant=Disabled  FdbkBlocksVariant=Forward  IdealPFdbkVariant=Disabled  SatFdbkVariant=Disabled  DerivativeFilterVariant=Disabled  NVariant=Disabled  NCopyVariant=Disabled_SignalSpec  FilterICVariant=Disabled  IntegratorICVariant=InternalICs  ExternalResetVariant=ExternalReset  TRSumVariant=Passthrough  SumFdbkVariant=Disabled  SumVariant=Sum_PI  TsampFilterVariant=InternalTs  TsampNgainVariant=Passthrough  TsampIntegralVariant=Passthrough  ExternalSaturationOutDataTypeStr=Inherit: Same as second input
  Error : Sum  Inputs=+-
  Error1 : Sum  Inputs=-+
  Error2 : Sum  Inputs=+-
  Memory : Memory
  Memory1 : Memory
  Memory2 : Memory
  MinMax : MinMax
  MinMax1 : MinMax
  MinMax2 : MinMax  Inputs=2
  OR : Logic  Operator=OR  AllPortsSameDT=off  OutDataTypeStr=boolean
  Product{,1..9} (10 alike) : Product
  Rate Transition : RateTransition  OutPortSampleTime=1/50
  Rate Transition1 : RateTransition  OutPortSampleTime=1/50
  Saturation1 : Saturate  UpperLimit=0  LowerLimit=-100
  Saturation2 : Saturate  UpperLimit=0  LowerLimit=-100
  Saturation3 : Saturate  UpperLimit=100  LowerLimit=0
  Saturation4 : Saturate  UpperLimit=100  LowerLimit=0
  Saturation8 : Saturate  UpperLimit=100  LowerLimit=-100
  Saturation9 : Saturate  UpperLimit=100  LowerLimit=-100
  Sum : Sum  Inputs=+++
  Sum1 : Sum  Inputs=+++
  Sum2 : Sum
  Sum3 : Sum  Inputs=-+
  Switch : Switch  Criteria=u2 > Threshold  SaturateOnIntegerOverflow=off  InputSameDT=off
  Switch1 : Switch  Criteria=u2 > Threshold  SaturateOnIntegerOverflow=off  InputSameDT=off
  Switch2 : Switch  Criteria=u2 > Threshold  SaturateOnIntegerOverflow=off  InputSameDT=off
  Target_Distance_Saturation : Saturate  UpperLimit=ACC_SensorMaxDistance  LowerLimit=2
  Terminator : Terminator
  Terminator1 : Terminator
  Terminator2 : Terminator
  Transfer Fcn First Order{4..11} (8 alike) : simulink/Discrete/Transfer Fcn First Order  PoleZ=0.9  ICPrevOutput=0.0  DoSatur=off
  Transfer Fcn First Order13 : simulink/Discrete/Transfer Fcn First Order  PoleZ=0.99  ICPrevOutput=0.0  DoSatur=off
  tACC_PID : Subsystem
  tag scope: ACC_Actual_Distance=global, ACC_Brake=global, ACC_Memory_Speed=global, ACC_PID_Output=global, ACC_Target_Distance=global, ACC_Target_Speed=global, ACC_Throttle=global, cACC_Brake_Demand=global, cACC_Throttle_Demand=global, tACC_Brake_Demand=global, tACC_PID_Output=global, tACC_Throttle_Demand=global
  wires:
  [ACC_Active] -> Product4/1
  MinMax1/1 -> Compare To Constant1/1
  Target_Distance_Saturation/1 -> [ACC_Target_Distance], Error1/1
  [Vehicle_Speed] -> Error/2
  [ACC_Active] -> Detect Increase/1, Product1/2, Product2/1
  Memory/1 -> Switch/3
  Error/1 -> Product1/1
  MinMax/1 -> Compare To Constant/1
  [SensorTargets_300000_ClosestTargetDistance] -> MinMax/1
  [Vehicle_Speed] -> Sum3/2
  Switch/1 -> Sum2/2
  Product1/1 -> ACC_PID/1  "difference betweer reference and actual speed"
  [ACC_Active] -> Compare To Zero/1
  Compare To Constant/1 -> Product2/2
  Compare To Constant1/1 -> Product4/2
  Compare To Zero/1 -> Product/2, Product5/1
  [Driver_Brake] -> Product/1
  [Driver_Throttle] -> Product5/2
  Sum1/1 -> Transfer Fcn First Order5/1
  Product5/1 -> Sum1/1
  ACC_PID/1 -> Product6/1
  Product6/1 -> Saturation2/1, Saturation3/1
  [ACC_Target_Speed] -> Error2/1
  [Vehicle_Speed] -> ACC_Speed_Distance_Gain/1(In1), Error2/2
  Saturation2/1 -> ACC_Brake_Gain1/1
  Saturation3/1 -> [cACC_Throttle_Demand]
  ACC_Brake_Gain1/1 -> [cACC_Brake_Demand]
  Product/1 -> Sum/3
  Saturation1/1 -> ACC_Brake_Gain2/1
  Saturation4/1 -> [tACC_Throttle_Demand]
  ACC_Brake_Gain2/1 -> [tACC_Brake_Demand]
  Discrete PID Controller1/1 -> Product9/1
  [cACC_Throttle_Demand] -> Sum1/2
  [cACC_Brake_Demand] -> Sum/2
  [tACC_Brake_Demand] -> Sum/1
  [tACC_Throttle_Demand] -> Sum1/3
  Product4/1 -> Product7/2, tACC_PID/2(In2), Product9/2, Discrete PID Controller1/2
  MinMax2/1 -> Saturation4/1, Saturation1/1, [tACC_PID_Output]
  Error2/1 -> Discrete PID Controller1/1
  Product9/1 -> MinMax2/1
  Product2/1 -> Product6/2, ACC_PID/2
  Transfer Fcn First Order5/1 -> Transfer Fcn First Order4/1
  Sum/1 -> Transfer Fcn First Order9/1
  Transfer Fcn First Order4/1 -> Transfer Fcn First Order6/1
  Transfer Fcn First Order6/1 -> Transfer Fcn First Order7/1
  Transfer Fcn First Order7/1 -> Saturation9/1
  Transfer Fcn First Order8/1 -> Transfer Fcn First Order10/1
  Transfer Fcn First Order9/1 -> Transfer Fcn First Order8/1
  Transfer Fcn First Order10/1 -> Transfer Fcn First Order11/1
  Transfer Fcn First Order11/1 -> Saturation8/1
  Saturation8/1 -> [ACC_Brake]
  Saturation9/1 -> [ACC_Throttle]
  Product7/1 -> MinMax2/2
  [SensorTargets_300000_ClosestTargetDistance] -> Transfer Fcn First Order13/1, MinMax1/1, Rate Transition/1
  Transfer Fcn First Order13/1 -> [ACC_Actual_Distance]
  ACC_Speed_Distance_Gain/1(Out1) -> Rate Transition1/1
  Error1/1 -> tACC_PID/1(In1)
  tACC_PID/1(Out1) -> [ACC_PID_Output], Product7/1
  [Additional_speed] -> Product3/1
  Detect Increase/1 -> Switch/2
  Product8/1 -> Switch1/3, [ACC_Target_Speed], Memory1/1
  Switch1/1 -> Memory/1, Error/1
  [reset_ACC] -> Detect Increase1/1
  [ACC_Memory_Speed] -> Switch1/1
  Detect Increase1/1 -> Switch1/2
  Rate Transition/1 -> Error1/2
  Rate Transition1/1 -> Target_Distance_Saturation/1
  Product3/1 -> Sum2/1
  ACC_Module_Activity_Flag/1 -> OR/1
  Sum2/1 -> Product8/1
  [ACC_Active] -> Product3/2
  [Driver_Throttle] -> ACC_PID/3
  [ACC_Active] -> Switch2/2
  Switch2/1 -> Memory2/1, [ACC_Memory_Speed]  "set speed memory"
  Memory1/1 -> Switch2/1
  Memory2/1 -> Switch2/3
  AP_Module_Activity_Flag/1 -> OR/2
  OR/1 -> Product8/2
  Sum3/1 -> Switch/1
  Constant/1 -> Sum3/1
  [ACC_Target_Distance] -> Terminator/1
  [ACC_Actual_Distance] -> Terminator1/1
  [ACC_PID_Output] -> Bus Creator/1
  [tACC_PID_Output] -> Bus Creator/2
  [tACC_Brake_Demand] -> Bus Creator/3
  [tACC_Throttle_Demand] -> Bus Creator/4
  Bus Creator/1 -> Terminator2/1

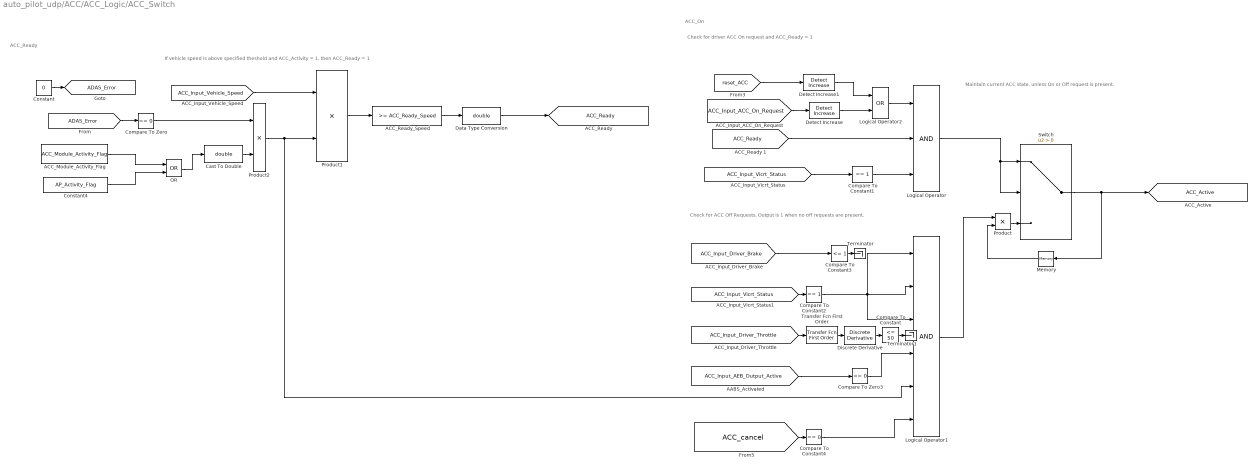
== system auto_pilot_udp/ACC/ACC_Logic/ACC_Switch ==
  note: ACC_On
  note: ACC_Ready
  note: If vehicle speed is above specified theshold and ACC_Activity = 1, then ACC_Ready = 1
  note: Check for driver ACC On request and ACC_Ready = 1
  note: Check for ACC Off Requests. Output is 1 when no off requests are present.
  note: Maintain current ACC state, unless On or Off request is present.
  ACC_Module_Activity_Flag : Constant  Value=ACC_Module_Activity_Flag
  ACC_Ready_Speed : simulink/Logic and Bit Operations/Compare To Constant  relop=>=  const=ACC_Ready_Speed  OutDataTypeStr=boolean
  Cast To Double : DataTypeConversion  OutDataTypeStr=double  SaturateOnIntegerOverflow=off  RndMeth=Floor
  Compare To Constant : simulink/Logic and Bit Operations/Compare To Constant  relop=<=  const=50  OutDataTypeStr=boolean
  Compare To Constant1 : simulink/Logic and Bit Operations/Compare To Constant  relop===  const=1  OutDataTypeStr=boolean
  Compare To Constant2 : simulink/Logic and Bit Operations/Compare To Constant  relop===  const=1  OutDataTypeStr=boolean
  Compare To Constant3 : simulink/Logic and Bit Operations/Compare To Constant  relop=<=  const=1  OutDataTypeStr=boolean
  Compare To Constant4 : simulink/Logic and Bit Operations/Compare To Constant  relop===  const=0  OutDataTypeStr=boolean
  Compare To Zero : simulink/Logic and Bit Operations/Compare To Zero  relop===  OutDataTypeStr=boolean
  Compare To Zero3 : simulink/Logic and Bit Operations/Compare To Zero  relop===  OutDataTypeStr=boolean
  Constant : Constant  Value=0
  Constant4 : Constant  Value=AP_Activity_Flag
  Data Type Conversion : DataTypeConversion  OutDataTypeStr=double  SaturateOnIntegerOverflow=off  RndMeth=Floor
  Detect Increase : simulink/Logic and Bit Operations/Detect Increase  vinit=0.0  OutDataTypeStr=boolean
  Detect Increase1 : simulink/Logic and Bit Operations/Detect Increase  vinit=0.0  OutDataTypeStr=boolean
  Discrete Derivative : simulink/Discrete/Discrete Derivative  gainval=1.0  ICPrevScaledInput=0.0  OutMin=[]  OutMax=[]  OutDataType=fixdt(1, 16)  OutScaling=2^-10  DoSatur=off
  Logical Operator : Logic  Inputs=3  AllPortsSameDT=off  OutDataTypeStr=boolean
  Logical Operator1 : Logic  Inputs=6  AllPortsSameDT=off  OutDataTypeStr=boolean
  Logical Operator2 : Logic  Operator=OR  AllPortsSameDT=off  OutDataTypeStr=boolean
  Memory : Memory
  OR : Logic  Operator=OR  AllPortsSameDT=off  OutDataTypeStr=boolean
  Product : Product
  Product1 : Product
  Product2 : Product
  Switch : Switch  Criteria=u2 > Threshold  SaturateOnIntegerOverflow=off  InputSameDT=off
  Terminator : Terminator
  Terminator1 : Terminator
  Transfer Fcn First Order : simulink/Discrete/Transfer Fcn First Order  PoleZ=0.99  ICPrevOutput=0.0  DoSatur=off
  tag scope: ACC_Active=global, ACC_Ready=global, ADAS_Error=global
  wires:
  Data Type Conversion/1 -> [ACC_Ready]
  [ACC_Input_Vehicle_Speed] -> Product1/1
  Product1/1 -> ACC_Ready_Speed/1
  ACC_Ready_Speed/1 -> Data Type Conversion/1
  Discrete Derivative/1 -> Compare To Constant/1
  Transfer Fcn First Order/1 -> Discrete Derivative/1
  Logical Operator/1 -> Switch/2, Switch/1
  Memory/1 -> Product/2
  Switch/1 -> [ACC_Active], Memory/1
  Compare To Constant2/1 -> Logical Operator1/1, Logical Operator1/3, Logical Operator1/2
  [ACC_Input_ACC_On_Request] -> Detect Increase/1
  [ACC_Input_Driver_Throttle] -> Transfer Fcn First Order/1
  Logical Operator1/1 -> Product/1
  [ACC_Input_Driver_Brake] -> Compare To Constant3/1
  [ACC_Input_Vicrt_Status] -> Compare To Constant2/1
  Product/1 -> Switch/3
  Detect Increase/1 -> Logical Operator2/2
  [ACC_Ready] -> Logical Operator/2
  [ACC_Input_AEB_Output_Active] -> Compare To Zero3/1
  Compare To Zero3/1 -> Logical Operator1/4
  [ACC_Input_Vicrt_Status] -> Compare To Constant1/1
  Compare To Constant1/1 -> Logical Operator/3
  [ADAS_Error] -> Compare To Zero/1
  Product2/1 -> Logical Operator1/5, Product1/2
  Compare To Zero/1 -> Product2/1
  [reset_ACC] -> Detect Increase1/1
  Detect Increase1/1 -> Logical Operator2/1
  Logical Operator2/1 -> Logical Operator/1
  ACC_Module_Activity_Flag/1 -> OR/1
  Constant4/1 -> OR/2
  OR/1 -> Cast To Double/1
  Cast To Double/1 -> Product2/2
  [ACC_cancel] -> Compare To Constant4/1
  Compare To Constant4/1 -> Logical Operator1/6
  Constant/1 -> [ADAS_Error]
  Compare To Constant3/1 -> Terminator/1
  Compare To Constant/1 -> Terminator1/1

== system auto_pilot_udp/ACC/ACC_Logic/ACC_Target_Acquisition ==
  SensorTargets_300000_ClosestTargetDistance : Subsystem
  SensorTargets_300000_ClosestTargetId : Subsystem
  SensorTargets_300000_InCurvedLane_mux : Subsystem
  SensorTargets_300000_InStraightLane_mux : Subsystem
  SensorTargets_300000_LateralDistance_mux : Subsystem
  SensorTargets_300000_LongitudinalDistance_mux : Subsystem

== system auto_pilot_udp/AEB/AEB_Logic/AEB_Brake_id  ==
  note: id of target with max brake demand
  Brake_Demand_max : Inport
  Brake_Demand_mux : Inport  Port=2
  Target_id_mux : Inport  Port=3
  MinMax3 : MinMax  Function=max
  No_Target_Display_Value : Constant  Value=No_Target_Display_Value
  Product5 : Product  OutDataTypeStr=double
  Relational Operator1 : RelationalOperator  Operator===  OutDataTypeStr=boolean  InputSameDT=off
  Switch4 : Switch  Criteria=u2 ~= 0  SaturateOnIntegerOverflow=off  InputSameDT=off
  Brake_Demand_max_id : Outport  VectorParamsAs1DForOutWhenUnconnected=off
  wires:
  MinMax3/1 -> Switch4/1
  Product5/1 -> MinMax3/1
  Relational Operator1/1 -> Product5/2
  Brake_Demand_max/1 -> Switch4/2, Relational Operator1/2
  Target_id_mux/1 -> Product5/1
  Brake_Demand_mux/1 -> Relational Operator1/1
  No_Target_Display_Value/1 -> Switch4/3
  Switch4/1 -> Brake_Demand_max_id/1

== system auto_pilot_udp/AEB/AEB_Logic/AEB_Trigger ==
  In1 : Inport
  In5 : Inport  Port=2
  In2 : Inport  Port=3
  In3 : Inport  Port=4
  In4 : Inport  Port=5
  AEB_Max_Speed : simulink/Logic and Bit Operations/Compare To Constant  relop=<  const=AEB_Max_Speed  OutDataTypeStr=boolean
  AEB_Steer_Max : simulink/Logic and Bit Operations/Compare To Constant  relop=<  const=AEB_Steer_Max*pi/180  OutDataTypeStr=boolean
  Abs2 : Abs  SaturateOnIntegerOverflow=off
  Compare To Pedestrian Type : simulink/Logic and Bit Operations/Compare To Constant  relop===  const=AEB_Pedestrian_type  OutDataTypeStr=boolean
  Constant : Constant
  Delay : Delay  DelayLength=1  InitialCondition=0
  Delay1 : Delay  InitialCondition=0
  Delay2 : Delay  DelayLength=3  InitialCondition=0
  Demux3 : Demux  Outputs=5
  Logical Operator : Logic  Inputs=7  AllPortsSameDT=off  OutDataTypeStr=boolean
  Mux3 : Mux  Inputs=5
  Product : Product  Inputs=4
  Rate Transition : RateTransition  OutPortSampleTime=1/AEB_Freq_Hz
  Rate Transition1 : RateTransition  OutPortSampleTime=1/AEB_Freq_Hz
  Rate Transition2 : RateTransition  OutPortSampleTime=1/AEB_Freq_Hz
  Switch : Switch  Criteria=u2 > Threshold  SaturateOnIntegerOverflow=off  InputSameDT=off
  AEB_Trigger : Outport  VectorParamsAs1DForOutWhenUnconnected=off
  wires:
  Logical Operator/1 -> AEB_Trigger/1
  In2/1 -> Mux3/2
  In3/1 -> Mux3/3
  In4/1 -> Mux3/4
  Product/1 -> Demux3/1
  Delay/1 -> Product/2
  In1/1 -> Mux3/1
  Demux3/4 -> Logical Operator/4
  [AEB_Input_Driver_Steering] -> Abs2/1
  Abs2/1 -> AEB_Steer_Max/1
  AEB_Steer_Max/1 -> Rate Transition/1
  In5/1 -> Mux3/5
  Demux3/5 -> Switch/3
  [AEB_Input_Vehicle_Speed] -> AEB_Max_Speed/1
  AEB_Max_Speed/1 -> Rate Transition1/1
  [AEB_Input_SensorTargets_type_mux] -> Rate Transition2/1
  Compare To Pedestrian Type/1 -> Switch/2
  Rate Transition2/1 -> Compare To Pedestrian Type/1
  Constant/1 -> Switch/1
  Delay1/1 -> Product/3
  Delay2/1 -> Product/4
  Rate Transition/1 -> Logical Operator/6
  Demux3/1 -> Logical Operator/1
  Demux3/3 -> Logical Operator/3
  Demux3/2 -> Logical Operator/2
  Switch/1 -> Logical Operator/5
  Rate Transition1/1 -> Logical Operator/7
  Mux3/1 -> Product/1, Delay/1, Delay2/1, Delay1/1

== system auto_pilot_udp/AEB/AEB_Logic/Distance_To_Collision_computation ==
  Distance : Inport
  Speed : Inport  Port=2
  ADAS_Control_Mode : Constant  Value=ADAS_Control_Mode
  AEB_Max_Decel : Constant  Value=AEB_Max_Decel(1)
  AEB_Max_Decel1 : Constant  Value=AEB_Max_Decel(2)
  Constant : Constant  Value=AEB_Min_Distance_at_Stop
  Gain : Gain  Gain=2
  Multiport Switch : MultiPortSwitch  Inputs=2  DataPortForDefault=Additional data port  DiagnosticForDefault=None  SaturateOnIntegerOverflow=off  InputSameDT=off
  Product1 : Product  Inputs=*/
  Rate Transition1 : RateTransition  OutPortSampleTime=1/AEB_Freq_Hz
  Square : Math  Operator=square  SignedPower=on
  Sum : Sum  Inputs=|++
  Distance_To_Collision_Current : Outport  VectorParamsAs1DForOutWhenUnconnected=off
  Distance_To_Collision_Threshold : Outport  Port=2  VectorParamsAs1DForOutWhenUnconnected=off
  wires:
  Multiport Switch/1 -> Gain/1
  Speed/1 -> Rate Transition1/1
  AEB_Max_Decel1/1 -> Multiport Switch/3
  ADAS_Control_Mode/1 -> Multiport Switch/1
  AEB_Max_Decel/1 -> Multiport Switch/2, Multiport Switch/4
  Product1/1 -> Sum/1
  Distance/1 -> Distance_To_Collision_Current/1
  Square/1 -> Product1/1
  Gain/1 -> Product1/2
  Rate Transition1/1 -> Square/1
  Sum/1 -> Distance_To_Collision_Threshold/1
  Constant/1 -> Sum/2

== system auto_pilot_udp/AEB/AEB_Logic/Target_XY_TimeToCollision ==
  Target_Y_Distance : Inport
  Target_X_Distance : Inport  Port=2
  "Target_Collision_Identifier_mux   " : Subsystem
  Target_X_TimeToCollision_mux : Subsystem
  Target_Y_TimeToCollision_mux : Subsystem
  Collision_Identifier : Outport  VectorParamsAs1DForOutWhenUnconnected=off
  wires:
  Target_X_Distance/1 -> Target_X_TimeToCollision_mux/1(Target_X_Distance)
  Target_Y_Distance/1 -> Target_Y_TimeToCollision_mux/1(Target_Y_Distance)
  "Target_Collision_Identifier_mux   "/1(Target_Collision_Identifier) -> Collision_Identifier/1
  Target_Y_TimeToCollision_mux/1(Target_Y_Left_TimeToCollision) -> "Target_Collision_Identifier_mux   "/1(Target_Y_Left_TimeToCollision)
  Target_Y_TimeToCollision_mux/2(Target_Y_Right_TimeToCollision) -> "Target_Collision_Identifier_mux   "/2(Target_Y_Right_TimeToCollision)
  Target_X_TimeToCollision_mux/1(Target_X_TimeToCollision) -> "Target_Collision_Identifier_mux   "/3(Target_X_TimeToCollision)

== system auto_pilot_udp/AEB/AEB_Logic/derivation_speed ==
  Distance : Inport
  Trigger : TriggerPort  VariantControl=Variant  PortDimensions=1
  Discrete Derivative : simulink/Discrete/Discrete Derivative  gainval=1.0  ICPrevScaledInput=0.0  OutMin=[]  OutMax=[]  OutDataType=fixdt(1, 16)  OutScaling=2^-10  DoSatur=off
  Gain : Gain  Gain=-1
  Speed_of_approaching : Outport
  wires:
  Distance/1 -> Discrete Derivative/1
  Discrete Derivative/1 -> Gain/1
  Gain/1 -> Speed_of_approaching/1
